simulink model "LogMoteur"  (R2021a)
settings: Solver=FixedStepAuto  StartTime=0.0  StopTime=5.5  FixedStep=1e-4  RelTol=1e-3
settings Model: Creator=rdelpoux  LastModifiedBy=rdelpoux
settings SolverCC: AlgebraicLoopSolver=TrustRegion

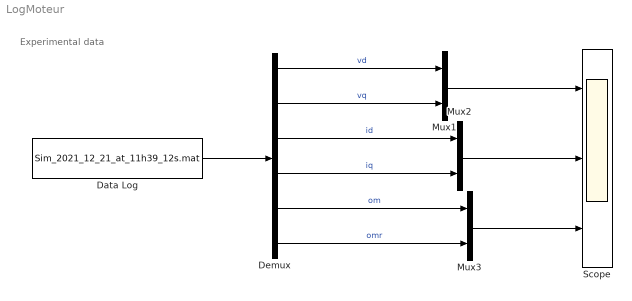
== system LogMoteur ==
  note: Experimental data
  Data Log : FromFile  FileName=Sim_2021_12_21_at_11h39_12s.mat  SampleTime=1e-4
  Demux : Demux  Outputs=6
  Mux1 : Mux  Inputs=2
  Mux2 : Mux  Inputs=2
  Mux3 : Mux  Inputs=2
  Scope : Scope  NumInputPorts=3
  wires:
  Data Log/1 -> Demux/1
  Demux/1 -> Mux1/1  "vd"
  Demux/2 -> Mux1/2  "vq"
  Demux/3 -> Mux2/1  "id"
  Demux/4 -> Mux2/2  "iq"
  Demux/5 -> Mux3/1  "om"
  Demux/6 -> Mux3/2  "omr"
  Mux1/1 -> Scope/1
  Mux2/1 -> Scope/2
  Mux3/1 -> Scope/3
